simulink model "ctrl_TT_ad_ctrl_cpp_ros_feedback_1"  (R2022b)
settings: Solver=FixedStepAuto  StartTime=0.0  StopTime=Tf  FixedStep=0.05  RelTol=1e-3
StopFcn:
  | save('testdata')
values from neighbouring files (symbols this model uses):
  adap = 1    [testdata.mat]
  Cp = [-70.34790039 18.70597267 -370.8000183 -33.25566673 18.72042656 -369.9571533 3.8263092 17.99342728 -368.5174255 40.77630615 14.78142262 -366.2670288 ... (183 elements, 3x61)]    [testdata.mat]
  Cp_prime = [4.4510680392 0.0017344668 0.1011438 4.44985762706 -0.08575700726 0.1715736104 4.43452754992 -0.37550053768 0.2668049284 4.4276356638 -0.45576590634 0.3213246444 ... (183 elements, 3x61)]    [testdata.mat]
  d = 250    [testdata.mat]
  Kp = 0.1    [testdata.mat]
  L1 =     [testdata.mat]
  Tf = 500    [testdata.mat]
  Ts = 0.05    [testdata.mat]
libraries: robotlib x30, sharedtransform x2, dspmathops x2
settings Model: Creator=yagkim  LastModifiedBy=vpetrov
settings SolverCC: AlgebraicLoopSolver=TrustRegion
settings OptimizationCC: EnhancedBackFolding=on  PassReuseOutputArgsAs=Individual arguments  ZeroExternalMemoryAtStartup=off  ZeroInternalMemoryAtStartup=off  MaxStackSize=64  OptimizeBlockOrder=speed  DifferentSizesBufferReuse=on  OptimizationCustomize=off  EfficientTunableParamExpr=on
settings DebuggingCC: ParameterTunabilityLossMsg=error  UnconnectedInputMsg=warning  UnconnectedOutputMsg=warning  UnconnectedLineMsg=warning  SFMachineParentedDataDiag=warning  ArithmeticOperatorsInVariantConditions=warning
settings HardwareCC: ProdBitPerPointer=32  ProdBitPerSizeT=32  ProdBitPerPtrDiffT=32  ProdLargestAtomicFloat=None  ProdIntDivRoundTo=Undefined  ProdEndianess=Unspecified  ProdWordSize=32  ProdHWDeviceType=Generic->Unspecified (assume 32-bit Generic)
settings ModelReferenceCC: EnableRefExpFcnMdlSchedulingChecks=on
settings SFSimCC: MATLABDynamicMemAlloc=off  CustomCodeUndefinedFunction=UseInterfaceOnly  SimTargetLang=C++
settings RTWCC: Description=Embedded Coder  SystemTargetFile=ert.tlc  HardwareBoard=Robot Operating System (ROS)  TLCOptions="-aInlineSetEventsForThisBaseRateFcn=TLC_FALSE -aSuppressMultiTaskScheduler=TLC_FALSE  -aRateBasedStepFcn=0"  TemplateMakefile=ert_default_tmf  GenerateReport=on  Toolchain=Catkin  LaunchReport=on  TargetLang=C++  DLArmComputeVersion=19.05
settings CodeAppCC: ForceParamTrailComments=on  IgnoreCustomStorageClasses=off  OperatorAnnotations=on  SimulinkDataObjDesc=on  SFDataObjDesc=on  InsertBlockDesc=on
settings ERTTargetCC: SupportContinuousTime=on

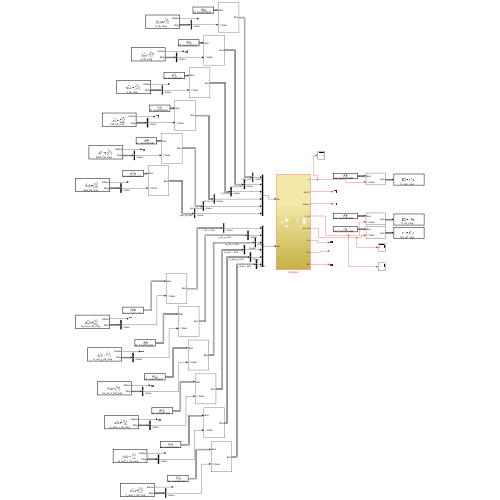
[thumbnail: Simulink's stored preview of the top-level diagram]
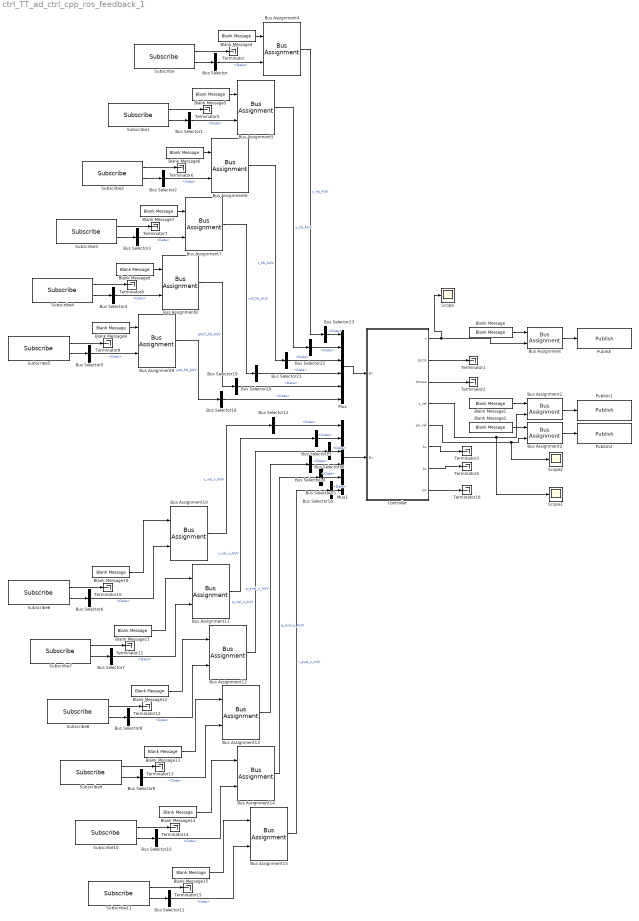
== system ctrl_TT_ad_ctrl_cpp_ros_feedback_1 ==
  Blank Message{,1..2,4..15} (15 alike) : robotlib/Blank Message  messageClass=Message  entityType=std_msgs/Float64  messageType=std_msgs/Float64  SampleTime=inf  legacyBusStruct=off
      settings: LibrarySourceBlock=roslib/ROS/Blank Message
  Bus Assignment{,1..2,4..15} (15 alike) : BusAssignment  AssignedSignals=Data
  Bus Selector{,1..23} (24 alike) : BusSelector  OutputSignals=Data
  Controller : Subsystem
  Mux : Mux  Inputs=6
  Mux1 : Mux  Inputs=6
  Publish : robotlib/Publish  topicSource=Specify your own  topic=/n_rpm_msg  messageType=std_msgs/Float64  legacyBusStruct=off  messageQueueLength=1
      settings: LibrarySourceBlock=roslib/ROS/Publish
  Publish1 : robotlib/Publish  topicSource=Specify your own  topic=/z_ref_msg  messageType=std_msgs/Float64  legacyBusStruct=off  messageQueueLength=1
      settings: LibrarySourceBlock=roslib/ROS/Publish
  Publish2 : robotlib/Publish  topicSource=Specify your own  topic=/psi_ref_msg  messageType=std_msgs/Float64  legacyBusStruct=off  messageQueueLength=1
      settings: LibrarySourceBlock=roslib/ROS/Publish
  Scope : Scope
  Scope1 : Scope
  Scope2 : Scope
  Subscribe : robotlib/Subscribe  topicSource=Specify your own  topic=/x_hb_msg  messageType=std_msgs/Float64  SampleTime=-1  legacyBusStruct=off  messageQueueLength=1
      settings: LibrarySourceBlock=roslib/ROS/Subscribe
  Subscribe1 : robotlib/Subscribe  topicSource=Specify your own  topic=/y_hb_msg  messageType=std_msgs/Float64  SampleTime=-1  legacyBusStruct=off  messageQueueLength=1
      settings: LibrarySourceBlock=roslib/ROS/Subscribe
  Subscribe10 : robotlib/Subscribe  topicSource=Specify your own  topic=/q_avel_y_hb_msg  messageType=std_msgs/Float64  SampleTime=-1  legacyBusStruct=off  messageQueueLength=1
      settings: LibrarySourceBlock=roslib/ROS/Subscribe
  Subscribe11 : robotlib/Subscribe  topicSource=Specify your own  topic=/r_avel_z_hb_msg  messageType=std_msgs/Float64  SampleTime=-1  legacyBusStruct=off  messageQueueLength=1
      settings: LibrarySourceBlock=roslib/ROS/Subscribe
  Subscribe2 : robotlib/Subscribe  topicSource=Specify your own  topic=/z_hb_msg  messageType=std_msgs/Float64  SampleTime=-1  legacyBusStruct=off  messageQueueLength=1
      settings: LibrarySourceBlock=roslib/ROS/Subscribe
  Subscribe3 : robotlib/Subscribe  topicSource=Specify your own  topic=/roll_hb_msg  messageType=std_msgs/Float64  SampleTime=-1  legacyBusStruct=off  messageQueueLength=1
      settings: LibrarySourceBlock=roslib/ROS/Subscribe
  Subscribe4 : robotlib/Subscribe  topicSource=Specify your own  topic=/pitch_hb_msg  messageType=std_msgs/Float64  SampleTime=-1  legacyBusStruct=off  messageQueueLength=1
      settings: LibrarySourceBlock=roslib/ROS/Subscribe
  Subscribe5 : robotlib/Subscribe  topicSource=Specify your own  topic=/yaw_hb_msg  messageType=std_msgs/Float64  SampleTime=-1  legacyBusStruct=off  messageQueueLength=1
      settings: LibrarySourceBlock=roslib/ROS/Subscribe
  Subscribe6 : robotlib/Subscribe  topicSource=Specify your own  topic=/u_vel_x_hb_msg  messageType=std_msgs/Float64  SampleTime=-1  legacyBusStruct=off  messageQueueLength=1
      settings: LibrarySourceBlock=roslib/ROS/Subscribe
  Subscribe7 : robotlib/Subscribe  topicSource=Specify your own  topic=/v_vel_y_hb_msg  messageType=std_msgs/Float64  SampleTime=-1  legacyBusStruct=off  messageQueueLength=1
      settings: LibrarySourceBlock=roslib/ROS/Subscribe
  Subscribe8 : robotlib/Subscribe  topicSource=Specify your own  topic=/w_vel_z_hb_msg  messageType=std_msgs/Float64  SampleTime=-1  legacyBusStruct=off  messageQueueLength=1
      settings: LibrarySourceBlock=roslib/ROS/Subscribe
  Subscribe9 : robotlib/Subscribe  topicSource=Specify your own  topic=/p_avel_x_hb_msg  messageType=std_msgs/Float64  SampleTime=-1  legacyBusStruct=off  messageQueueLength=1
      settings: LibrarySourceBlock=roslib/ROS/Subscribe
  Terminator{,1..16} (17 alike) : Terminator
  wires:
  Bus Assignment4/1 -> Bus Selector23/1  "x_hb_AUV"
  Bus Assignment6/1 -> Bus Selector21/1  "z_hb_AUV"
  Bus Assignment7/1 -> Bus Selector20/1  "roll_hb_AUV"
  Bus Assignment8/1 -> Bus Selector19/1  "pitch_hb_AUV"
  Bus Assignment9/1 -> Bus Selector18/1  "yaw_hb_AUV"
  Mux/1 -> Controller/1(Bx)
  Mux1/1 -> Controller/2(Bv)
  Bus Assignment11/1 -> Bus Selector13/1  "v_vel_y_AUV"
  Bus Assignment12/1 -> Bus Selector17/1  "w_vel_z_AUV"
  Bus Assignment13/1 -> Bus Selector14/1  "p_avel_x_AUV"
  Bus Assignment14/1 -> Bus Selector15/1  "q_avel_y_AUV"
  Bus Assignment15/1 -> Bus Selector16/1  "r_avel_z_AUV"
  Controller/1(n) -> Scope/1, Bus Assignment/2
  Controller/4(z_ref) -> Scope1/1, Bus Assignment1/2
  Controller/5(psi_ref) -> Scope2/1, Bus Assignment2/2
  Controller/6(bv) -> Terminator3/1
  Controller/7(bx) -> Terminator4/1
  Bus Assignment/1 -> Publish/1
  Blank Message/1 -> Bus Assignment/1
  Blank Message1/1 -> Bus Assignment1/1
  Bus Assignment1/1 -> Publish1/1
  Blank Message2/1 -> Bus Assignment2/1
  Bus Assignment2/1 -> Publish2/1
  Subscribe/1 -> Terminator/1
  Bus Selector/1 -> Bus Assignment4/2  "<Data>"
  Subscribe/2 -> Bus Selector/1
  Blank Message4/1 -> Bus Assignment4/1
  Subscribe1/1 -> Terminator5/1
  Bus Selector1/1 -> Bus Assignment5/2  "<Data>"
  Blank Message5/1 -> Bus Assignment5/1
  Subscribe1/2 -> Bus Selector1/1
  Bus Assignment5/1 -> Bus Selector22/1  "y_hb_AUV"
  Blank Message6/1 -> Bus Assignment6/1
  Bus Selector2/1 -> Bus Assignment6/2  "<Data>"
  Subscribe2/2 -> Bus Selector2/1
  Subscribe2/1 -> Terminator6/1
  Blank Message7/1 -> Bus Assignment7/1
  Bus Selector3/1 -> Bus Assignment7/2  "<Data>"
  Subscribe3/2 -> Bus Selector3/1
  Subscribe3/1 -> Terminator7/1
  Blank Message8/1 -> Bus Assignment8/1
  Bus Selector4/1 -> Bus Assignment8/2  "<Data>"
  Subscribe4/2 -> Bus Selector4/1
  Subscribe4/1 -> Terminator8/1
  Bus Selector5/1 -> Bus Assignment9/2  "<Data>"
  Subscribe5/2 -> Bus Selector5/1
  Blank Message9/1 -> Bus Assignment9/1
  Subscribe5/1 -> Terminator9/1
  Bus Selector6/1 -> Bus Assignment10/2  "<Data>"
  Subscribe6/2 -> Bus Selector6/1
  Blank Message10/1 -> Bus Assignment10/1
  Subscribe6/1 -> Terminator10/1
  Bus Assignment10/1 -> Bus Selector12/1  "u_vel_x_AUV"
  Bus Selector7/1 -> Bus Assignment11/2  "<Data>"
  Blank Message11/1 -> Bus Assignment11/1
  Subscribe7/2 -> Bus Selector7/1
  Subscribe7/1 -> Terminator11/1
  Bus Selector8/1 -> Bus Assignment12/2  "<Data>"
  Blank Message12/1 -> Bus Assignment12/1
  Subscribe8/2 -> Bus Selector8/1
  Subscribe8/1 -> Terminator12/1
  Bus Selector9/1 -> Bus Assignment13/2  "<Data>"
  Blank Message13/1 -> Bus Assignment13/1
  Subscribe9/2 -> Bus Selector9/1
  Subscribe9/1 -> Terminator13/1
  Bus Selector10/1 -> Bus Assignment14/2  "<Data>"
  Blank Message14/1 -> Bus Assignment14/1
  Subscribe10/2 -> Bus Selector10/1
  Subscribe10/1 -> Terminator14/1
  Bus Selector11/1 -> Bus Assignment15/2  "<Data>"
  Blank Message15/1 -> Bus Assignment15/1
  Subscribe11/2 -> Bus Selector11/1
  Subscribe11/1 -> Terminator15/1
  Bus Selector12/1 -> Mux1/1  "<Data>"
  Bus Selector13/1 -> Mux1/2  "<Data>"
  Bus Selector14/1 -> Mux1/4  "<Data>"
  Bus Selector15/1 -> Mux1/5  "<Data>"
  Bus Selector16/1 -> Mux1/6  "<Data>"
  Bus Selector17/1 -> Mux1/3  "<Data>"
  Bus Selector18/1 -> Mux/6  "<Data>"
  Bus Selector19/1 -> Mux/5  "<Data>"
  Bus Selector20/1 -> Mux/4  "<Data>"
  Bus Selector21/1 -> Mux/3  "<Data>"
  Bus Selector22/1 -> Mux/2  "<Data>"
  Bus Selector23/1 -> Mux/1  "<Data>"
  Controller/2(dLCG) -> Terminator1/1
  Controller/3(dmass) -> Terminator2/1
  Controller/8(dX) -> Terminator16/1

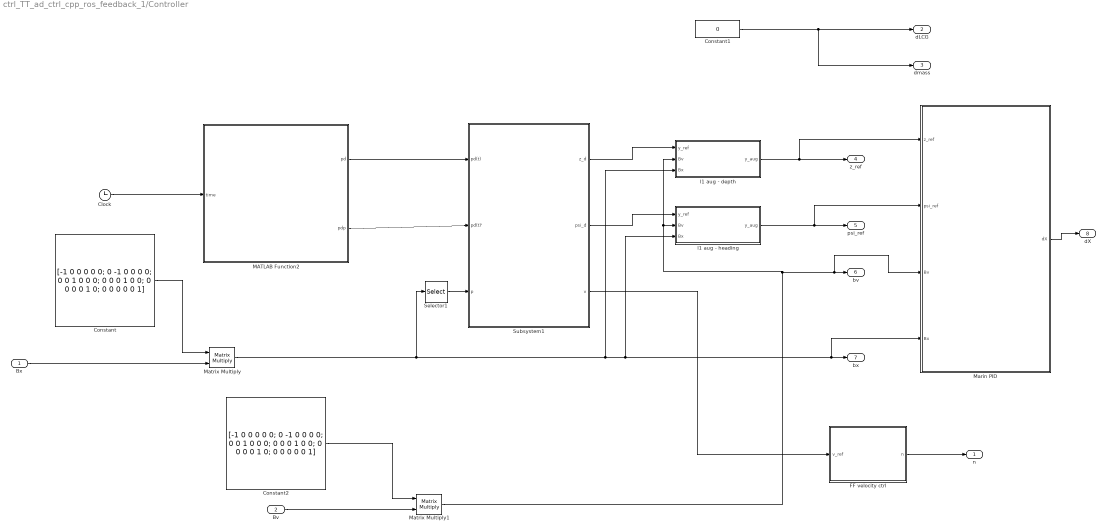
== system ctrl_TT_ad_ctrl_cpp_ros_feedback_1/Controller ==
  Bx : Inport
  Bv : Inport  Port=2
  Clock : Clock
  Constant : Constant  Value=[-1 0 0 0 0 0; 0 -1 0 0 0 0; 0 0 1 0 0 0; 0 0 0 1 0 0; 0 0 0 0 1 0; 0 0 0 0 0 1]
  Constant1 : Constant  Value=0
  Constant2 : Constant  Value=[-1 0 0 0 0 0; 0 -1 0 0 0 0; 0 0 1 0 0 0; 0 0 0 1 0 0; 0 0 0 0 1 0; 0 0 0 0 0 1]
  FF velocity ctrl : MATLAB Function  TreatAsAtomicUnit=on
  MATLAB Function2 : MATLAB Function  TreatAsAtomicUnit=on
  Marin PID : MATLAB Function  TreatAsAtomicUnit=on
  Matrix Multiply : Product  Multiplication=Matrix(*)
  Matrix Multiply1 : Product  Multiplication=Matrix(*)
  Selector1 : Selector  InputPortWidth=6  IndexOptions=Index vector (dialog)  Indices=[1 2 3]  OutputSizes=1
  Subsystem1 : Subsystem
  l1 aug - depth : MATLAB Function  TreatAsAtomicUnit=on
  l1 aug - heading : MATLAB Function  TreatAsAtomicUnit=on
  n : Outport
  dLCG : Outport  Port=2
  dmass : Outport  Port=3
  z_ref : Outport  Port=4
  psi_ref : Outport  Port=5
  bv : Outport  Port=6
  bx : Outport  Port=7
  dX : Outport  Port=8
  wires:
  FF velocity ctrl/1(n) -> n/1
  Subsystem1/3(v) -> FF velocity ctrl/1(v_ref)
  Constant1/1 -> dLCG/1, dmass/1
  MATLAB Function2/1(pd) -> Subsystem1/1(pd(t))
  MATLAB Function2/2(pdp) -> Subsystem1/2(pd(t)')
  Bx/1 -> Matrix Multiply/2
  Selector1/1 -> Subsystem1/3(p)
  Clock/1 -> MATLAB Function2/1(time)
  Matrix Multiply/1 -> Selector1/1, l1 aug - depth/3(Bx), Marin PID/4(Bx), bx/1, l1 aug - heading/3(Bx)
  Constant/1 -> Matrix Multiply/1
  Bv/1 -> Matrix Multiply1/2
  Matrix Multiply1/1 -> l1 aug - depth/2(Bv), l1 aug - heading/2(Bv), Marin PID/3(Bv), bv/1
  Constant2/1 -> Matrix Multiply1/1
  l1 aug - depth/1(y_aug) -> Marin PID/1(z_ref), z_ref/1
  l1 aug - heading/1(y_aug) -> Marin PID/2(psi_ref), psi_ref/1
  Subsystem1/1(z_d) -> l1 aug - depth/1(y_ref)
  Subsystem1/2(psi_d) -> l1 aug - heading/1(y_ref)
  Marin PID/1(dX) -> dX/1

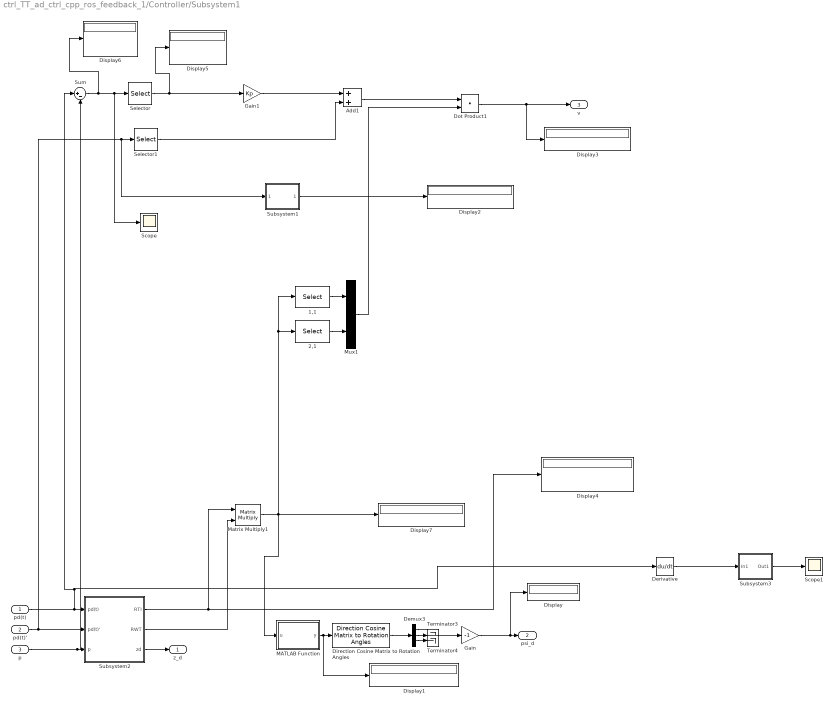
== system ctrl_TT_ad_ctrl_cpp_ros_feedback_1/Controller/Subsystem1 ==
  pd(t) : Inport
  pd(t)' : Inport  Port=2
  p : Inport  Port=3
  1,1 : Selector  NumberOfDimensions=2  InputPortWidth=3  IndexOptions=Index vector (dialog),Index vector (dialog)  Indices=1,1  OutputSizes=1,1
  2,1 : Selector  NumberOfDimensions=2  InputPortWidth=3  IndexOptions=Index vector (dialog),Index vector (dialog)  Indices=2,1  OutputSizes=1,1
  Add1 : Sum
  Demux3 : Demux  Outputs=3
  Derivative : Derivative
  Direction Cosine Matrix to Rotation Angles : sharedtransform/Direction Cosine Matrix to Rotation Angles  rotationOrder=ZYX  aMode=aMode  action=None  tolerance=eps(2)
      settings: LibrarySourceBlock=|
      | aerolibtransform2/Direction Cosine Matrix
      | to Rotation Angles
  Display{,1..7} (8 alike) : Display
  Dot Product1 : DotProduct  OutDataTypeStr=Inherit: Inherit via internal rule
  Gain : Gain  Gain=-1
  Gain1 : Gain  Gain=Kp
  MATLAB Function : MATLAB Function  TreatAsAtomicUnit=on
  Matrix Multiply1 : Product  Multiplication=Matrix(*)
  Mux1 : Mux  Inputs=2
  Scope : Scope
  Scope1 : Scope
  Selector : Selector  InputPortWidth=3  IndexOptions=Index vector (dialog)  Indices=[1 2]  OutputSizes=1
  Selector1 : Selector  InputPortWidth=3  IndexOptions=Index vector (dialog)  Indices=[1 2]  OutputSizes=1
  Subsystem1 : Subsystem
  Subsystem2 : Subsystem
  Subsystem3 : Subsystem
  Sum : Sum  Inputs=|+-
  Terminator3 : Terminator
  Terminator4 : Terminator
  z_d : Outport
  psi_d : Outport  Port=2
  v : Outport  Port=3
  wires:
  pd(t)'/1 -> Subsystem2/2(pd(t)'), Subsystem1/1(pd(t)'), Selector1/1
  pd(t)/1 -> Derivative/1, Sum/1, Subsystem2/1(pd(t))
  p/1 -> Sum/2, Subsystem2/3(p)
  Subsystem2/1(RTI) -> Matrix Multiply1/1, Display4/1
  2,1/1 -> Mux1/2
  1,1/1 -> Mux1/1
  Subsystem2/3(zd) -> z_d/1
  Gain/1 -> Display/1, psi_d/1
  Subsystem2/2(RWT) -> Matrix Multiply1/2
  Sum/1 -> Display6/1, Scope/1, Selector/1
  Derivative/1 -> Subsystem3/1(In1)
  Subsystem3/1(Out1) -> Scope1/1
  Gain1/1 -> Add1/1
  Add1/1 -> Dot Product1/1
  Mux1/1 -> Dot Product1/2
  Dot Product1/1 -> Display3/1, v/1
  Selector/1 -> Display5/1, Gain1/1
  Selector1/1 -> Add1/2
  Subsystem1/1(Out1) -> Display2/1
  Direction Cosine Matrix to Rotation Angles/1 -> Demux3/1
  Matrix Multiply1/1 -> MATLAB Function/1(u), Display7/1, 2,1/1, 1,1/1
  MATLAB Function/1(y) -> Display1/1, Direction Cosine Matrix to Rotation Angles/1
  Demux3/2 -> Terminator3/1
  Demux3/3 -> Terminator4/1
  Demux3/1 -> Gain/1

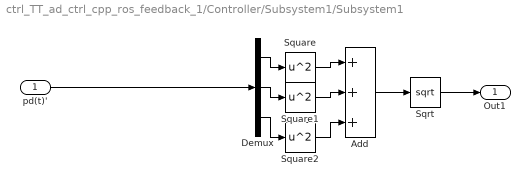
== system ctrl_TT_ad_ctrl_cpp_ros_feedback_1/Controller/Subsystem1/Subsystem1 ==
  pd(t)' : Inport
  Add : Sum  Inputs=+++
  Demux : Demux  Outputs=3
  Sqrt : Sqrt
  Square : Math  Operator=square
  Square1 : Math  Operator=square
  Square2 : Math  Operator=square
  Out1 : Outport
  wires:
  Square2/1 -> Add/3
  Demux/3 -> Square2/1
  pd(t)'/1 -> Demux/1
  Demux/1 -> Square/1
  Demux/2 -> Square1/1
  Add/1 -> Sqrt/1
  Square/1 -> Add/1
  Square1/1 -> Add/2
  Sqrt/1 -> Out1/1

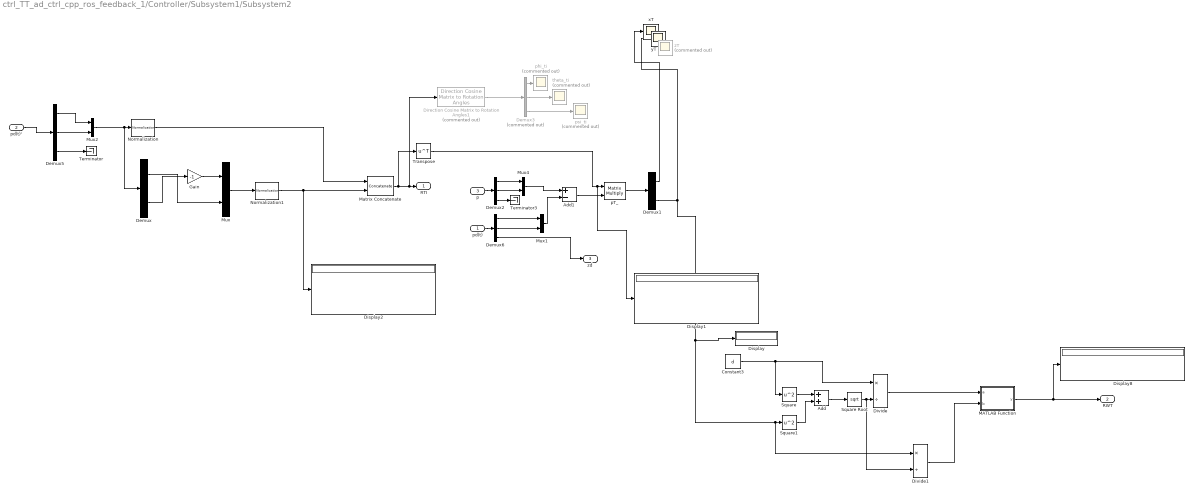
== system ctrl_TT_ad_ctrl_cpp_ros_feedback_1/Controller/Subsystem1/Subsystem2 ==
  pd(t) : Inport
  pd(t)' : Inport  Port=2
  p : Inport  Port=3
  Add : Sum
  Add1 : Sum  Inputs=+-
  Constant3 : Constant  Value=d
  Demux : Demux  Outputs=2
  Demux1 : Demux  Outputs=2
  Demux2 : Demux  Outputs=3
  Demux3 : Demux  Commented=on  Outputs=3
  Demux5 : Demux  Outputs=3
  Demux6 : Demux  Outputs=3
  Direction Cosine Matrix to Rotation Angles1 : sharedtransform/Direction Cosine Matrix to Rotation Angles  Commented=on  rotationOrder=XYZ  aMode=aMode  action=None  tolerance=eps(2)
  Display{,1..2,8} (4 alike) : Display
  Divide : Product  Inputs=*/
  Divide1 : Product  Inputs=*/
  Gain : Gain  Gain=-1
  MATLAB Function : MATLAB Function  TreatAsAtomicUnit=on
  Matrix Concatenate : Concatenate  Mode=Multidimensional array  ConcatenateDimension=2
  Mux{,1..2,4} (4 alike) : Mux  Inputs=2
  Normalization : dspmathops/Normalization  NormType=2-norm  Bias=1e-10  NormOver=Each column  Dimension=1  roundingMode=Floor  overflowMode=off  accumDataTypeStr=Inherit: Same as product output  accumLastDataTypeStr=Inherit: Same as product output  outputDataTypeStr=Inherit: Same as product output  outputMin=[]  outputMax=[]  outputLastDataTypeStr=Inherit: Same as product output
  Normalization1 : dspmathops/Normalization  NormType=2-norm  Bias=1e-10  NormOver=Each column  Dimension=1  roundingMode=Floor  overflowMode=off  accumDataTypeStr=Inherit: Same as product output  accumLastDataTypeStr=Inherit: Same as product output  outputDataTypeStr=Inherit: Same as product output  outputMin=[]  outputMax=[]  outputLastDataTypeStr=Inherit: Same as product output
  Square : Math  Operator=square
  Square Root : Sqrt
  Square1 : Math  Operator=square
  Terminator : Terminator
  Terminator3 : Terminator
  Transpose : Math  Operator=transpose
  pT_ : Product  Multiplication=Matrix(*)
  phi_ti : Scope  Commented=on
  psi_ti : Scope  Commented=on
  theta_ti : Scope  Commented=on
  xT : Scope
  yT : Scope
  zT : Scope  Commented=on
  RTI : Outport
  RWT : Outport  Port=2
  zd : Outport  Port=3
  wires:
  Gain/1 -> Mux/1
  Demux/2 -> Gain/1
  Demux/1 -> Mux/2
  Mux/1 -> Normalization1/1
  Normalization/1 -> Matrix Concatenate/1
  Normalization1/1 -> Matrix Concatenate/2, Display2/1
  Matrix Concatenate/1 -> Direction Cosine Matrix to Rotation Angles1/1, RTI/1, Transpose/1
  Transpose/1 -> Display1/1, pT_/1
  Add1/1 -> pT_/2
  pT_/1 -> Demux1/1
  Demux1/2 -> yT/1, Display/1, Divide1/1, Square1/1
  Demux1/1 -> xT/1
  Direction Cosine Matrix to Rotation Angles1/1 -> Demux3/1
  Demux3/3 -> psi_ti/1
  Demux3/2 -> theta_ti/1
  Demux3/1 -> phi_ti/1
  Constant3/1 -> Square/1, Divide/1
  Square Root/1 -> Divide1/2, Divide/2
  Add/1 -> Square Root/1
  Square/1 -> Add/1
  Square1/1 -> Add/2
  Divide/1 -> MATLAB Function/1(a)
  Divide1/1 -> MATLAB Function/2(b)
  MATLAB Function/1(y) -> RWT/1, Display8/1
  Demux6/3 -> zd/1
  pd(t)'/1 -> Demux5/1
  Mux2/1 -> Demux/1, Normalization/1
  Demux5/1 -> Mux2/1
  Demux5/2 -> Mux2/2
  Demux5/3 -> Terminator/1
  Demux2/1 -> Mux4/1
  Demux2/3 -> Terminator3/1
  Demux2/2 -> Mux4/2
  Mux4/1 -> Add1/1
  p/1 -> Demux2/1
  Demux6/1 -> Mux1/1
  Demux6/2 -> Mux1/2
  pd(t)/1 -> Demux6/1
  Mux1/1 -> Add1/2

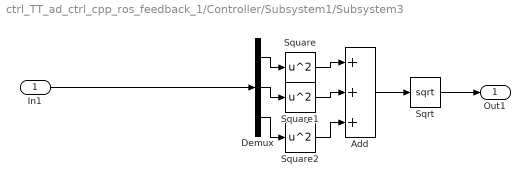
== system ctrl_TT_ad_ctrl_cpp_ros_feedback_1/Controller/Subsystem1/Subsystem3 ==
  In1 : Inport
  Add : Sum  Inputs=+++
  Demux : Demux  Outputs=3
  Sqrt : Sqrt
  Square : Math  Operator=square
  Square1 : Math  Operator=square
  Square2 : Math  Operator=square
  Out1 : Outport
  wires:
  Sqrt/1 -> Out1/1
  Square1/1 -> Add/2
  Square/1 -> Add/1
  Add/1 -> Sqrt/1
  Demux/2 -> Square1/1
  Demux/1 -> Square/1
  In1/1 -> Demux/1
  Demux/3 -> Square2/1
  Square2/1 -> Add/3

== matlab function ctrl_TT_ad_ctrl_cpp_ros_feedback_1/Controller/FF velocity ctrl ==
  settings: updateMethod=DISCRETE
  data: v_ref input; n output
function n   = fcn(v_ref)




KP_n = 5;
FF_inv = 4;



%% Prop
n = v_ref/FF_inv;

== matlab function ctrl_TT_ad_ctrl_cpp_ros_feedback_1/Controller/l1 aug - heading ==
  settings: updateMethod=DISCRETE
  data: y_ref input; Bv input; Bx input; y_aug output; Ts parameter; adap parameter; L1 parameter
function y_aug    = fcn(y_ref,Bv,Bx,Ts,adap,L1)
%pd,NomegaNI,

persistent xu xd


%% Variables for feedback
x = Bx(1); y = Bx(2); z = Bx(3); phi = Bx(4); theta = Bx(5); psi = Bx(6);
p = [x;y;z];
uN = Bv(1); vN = Bv(2); wN = Bv(3); pB = Bv(4); qB=Bv(5); rB = Bv(6);
uB = -uN; vB = -vN; wB = wN;

%% Control Parameters  
% Gains for PF augmentation
Ts = Ts;
Am = L1.Amz; Bm = L1.Bmz; Cm = L1.Cmz; 
Phiinv = L1.Phiinvz; Lambda = L1.Lambdaz;
Ao = L1.Aoz; Bo = L1.Boz; Co = L1.Coz;

%% Output Definition
y = psi;;

%% Initialize
if isempty(xu)
        xu = zeros(length(Ao),1);
        xd = Cm'*inv(Cm*Cm')*y;
        xu_next = xu;
        xd_next = xd;
end



%% L1 Augmentation - dive

if adap 

    yd = Cm*xd;
    vec1    =   [eye(size(Bm,2)); zeros(size(Am,1)-size(Bm,2),size(Bm,2))];
    sigma = -Phiinv*expm(Lambda*(Am/Lambda)*Ts)*vec1*(yd-y);

    xu_next = expm(Ao*Ts)*xu + inv(Ao)*(expm(Ao*Ts)-eye(length(Bo)))*(Bo*expm(-Am*Ts)*sigma);
    Kg = -inv(Cm*inv(Am)*Bm);
    ud = Kg*y_ref - Co*xu;

    xd_next = expm(Am*Ts)*xd + inv(Am)*(expm(Am*Ts)-eye(length(Am)))*(Bm*ud + sigma);

    y_aug = ud;

else 

    y_aug = y_ref;

    xd_next = xd;
    xu_next = xu;

end




%% Save variables for next loop
xu = xu_next;
xd = xd_next;

== matlab function ctrl_TT_ad_ctrl_cpp_ros_feedback_1/Controller/l1 aug - depth ==
  settings: updateMethod=DISCRETE
  data: y_ref input; Bv input; Bx input; y_aug output; Ts parameter; adap parameter; L1 parameter
function y_aug    = fcn(y_ref,Bv,Bx,Ts,adap,L1)
%pd,NomegaNI,

persistent xu xd


%% Variables for feedback
x = Bx(1); y = Bx(2); z = Bx(3); phi = Bx(4); theta = Bx(5); psi = Bx(6);
p = [x;y;z];
uN = Bv(1); vN = Bv(2); wN = Bv(3); pB = Bv(4); qB=Bv(5); rB = Bv(6);
uB = -uN; vB = -vN; wB = wN;

%% Control Parameters  
% Gains for PF augmentation
Ts = Ts;
Am = L1.Amz; Bm = L1.Bmz; Cm = L1.Cmz; 
Phiinv = L1.Phiinvz; Lambda = L1.Lambdaz;
Ao = L1.Aoz; Bo = L1.Boz; Co = L1.Coz;
%% Output Definition
y = z; 

%% Initialize
if isempty(xu)
        xu = zeros(length(Ao),1);
        xd = Cm'*inv(Cm*Cm')*y;
        xu_next = xu;
        xd_next = xd;
end



%% L1 Augmentation - dive

if adap 

    yd = Cm*xd;
    vec1    =   [eye(size(Bm,2)); zeros(size(Am,1)-size(Bm,2),size(Bm,2))];
    sigma = -Phiinv*expm(Lambda*(Am/Lambda)*Ts)*vec1*(yd-y);

    xu_next = expm(Ao*Ts)*xu + inv(Ao)*(expm(Ao*Ts)-eye(length(Bo)))*(Bo*expm(-Am*Ts)*sigma);
    Kg = -inv(Cm*inv(Am)*Bm);
    ud = Kg*y_ref - Co*xu;

    xd_next = expm(Am*Ts)*xd + inv(Am)*(expm(Am*Ts)-eye(length(Am)))*(Bm*ud + sigma);

    y_aug = ud;

else 

    y_aug = y_ref;

    xd_next = xd;
    xu_next = xu;

end




%% Save variables for next loop
xu = xu_next;
xd = xd_next;

== matlab function ctrl_TT_ad_ctrl_cpp_ros_feedback_1/Controller/Subsystem1/MATLAB Function ==
  data: u input; y output
function y = R3(u)

y = [u(1,1) u(1,2) 0; u(2,1) u(2,2) 0; 0 0 1];

== matlab function ctrl_TT_ad_ctrl_cpp_ros_feedback_1/Controller/MATLAB Function2 ==
  data: time input; pd output; pdp output; Cp_prime parameter; Cp parameter; Tf parameter
function [pd, pdp] = fcn(time, Cp_prime, Cp, Tf)




pd = BernsteinPoly(Cp,time,0,Tf);
pdp = BernsteinPoly(Cp_prime,time,0,Tf);

% pd = [gamma; gamma/2 ; -50];
% 
% 
% pdp = [1 ; 1/2; 0];

end










function  poly_t  = BernsteinPoly(Cp,t,t0,tf)

% INPUTS:
% Cp is a matrix n by N+1 (n: dimension of polynomial, N: order of polynomial) 
% t is a time vector
% OUTPUT:
% poly_t: n-dimensional polynomial evaluated at each time t

% if t is a scalar, it returns the value of Bernstein Poly at t in [t0,tf]
% if t0 and tf are not provided, it returns the value of Bernstein Poly at t in [0,1]

% Written by: Venanzio Cichella       

%%%%%%%%%%%%%%%%%%%%%%%%%%%%%%%%%%%%%%%%%%%%%%

coder.extrinsic('exist')

[~, N] = size(Cp);
N = N-1;


% if length(t) > 1
%     B = BernsteinMatrix_a2b(N,t)';
%     poly_t = Cp*B;
% else
%     if ~exist('t0','var')
%         B = BernsteinMatrix_a2b(N,t)';
%         poly_t = Cp*B;
%     else
%         B = BernsteinMatrix_a2b(N,t,t0,tf)';
%         poly_t = Cp*B;
%     end
% end
B = BernsteinMatrix_a2b(N,t,t0,tf)';
poly_t = Cp*B;


end










function b = BernsteinMatrix_a2b(N, t, tmin, tmax)

% Inputs: order N, time vector t = [t0 ... tm], no need for tmin and tmax.
% Output: b = [b0N(t0) b1N(t0) ... bNN(t0);
%              b0N(t1) b1N(t1) ... bNN(t1);
%              ...
%              b0N(tm) b1N(tm) ... bNN(tm);
% Use: If Cp is a row vector of N+1 control points,
%       the Nth order Bezier curve is given by xN=Cp*b';
% This function is used in BernsteinPoly

% Alternatively
% Inputs: order n, scalar time t', tmin and tmax
% Output: b = [b0n(t') b1n(t') ... bnn(t')]
% Use: If Cp is a row vector of N+1 control points,
%       the Nth order Bezier curve evaluated at t' is given by xn=Cp*b';
% Comment: This is more efficient but not as robust as de Casteljau
%           It works best for low-order curves

% Written by: Venanzio Cichella       

%%%%%%%%%%%%%%%%%%%%%%%%%%%%%%%%%%%%%%%%%%%%%%

if length(t) > 1
    tmax = t(length(t));
    tmin = t(1);
end
%coder.extrinsic('exist')
%if ~exist('tmin','var')
%    tmin = 0; tmax = 1;
%end



% compute B(j+1) = binomial(n, j), j = 0..n
t = t';
B = ones(N+1, 1); 
for j = 1:ceil(N/2)
  B(j+1) = B(j)*(N+1-j)/j;
  B(N+1-j) = B(j+1);
end
% compute T(i, j) = (t(i)-tmin)^j, TT(i, j) = (tmax-t(i))^(N-j)
T = ones(length(t), N+1);
TT = ones(length(t), N+1);
% turn a row t into a column t so that 
% we can do diag(t)*T(:,j) by t.*T(:,j)
tp = reshape(t, length(t), 1)-tmin;
ttp = tmax - t;
% Compute binomial(N, j)*(t(i)-tmin)^j*(tmax-t(i))^(N-j)
for j = 1:N 
  T(:, j+1) = tp .* T(:, j); 
  T(:, j) = T(:, j) .* B(j);
 TT(:,N+1-j) = ttp .* TT(:,N+2-j);
end

% Compute binomial(N, j)*(t(i)-tmin)^j*(tmax-t(i))^(N-j)/((tmax-tmin)^N)
b =  T.*TT./((tmax-tmin)^N);

end

== matlab function ctrl_TT_ad_ctrl_cpp_ros_feedback_1/Controller/Subsystem1/Subsystem2/MATLAB Function ==
  data: a input; y output; b input
function y = fcn(a,b)

%y = [a,b,0;-b,a,0;0,0,1];
y = [a,b;-b,a];

== matlab function ctrl_TT_ad_ctrl_cpp_ros_feedback_1/Controller/Marin PID ==
  settings: updateMethod=DISCRETE
  data: z_ref input; psi_ref input; Bv input; Bx input; dX output; Ts parameter
function dX   = fcn(z_ref,psi_ref,Bv,Bx,Ts)

persistent zerr_prev zerr_int_prev thetaerr_prev thetaerr_int_prev psierr_prev psierr_int_prev

%% Initialize
if isempty(zerr_prev)
        zerr_prev = 0;
        zerr_int_prev = 0;
        thetaerr_prev = 0;
        thetaerr_int_prev = 0;
        psierr_prev = 0;
        psierr_int_prev = 0;
end


%% Variables for feedback
x = Bx(1); y = Bx(2); z = Bx(3); phi = Bx(4); theta = Bx(5); psi = Bx(6);
p = [x;y;z];
uN = Bv(1); vN = Bv(2); wN = Bv(3); pB = Bv(4); qB=Bv(5); rB = Bv(6);
uB = -uN; vB = -vN; wB = wN;


%% Gains
KP_APz = 3;
KI_APz = 0*0.1044;
KD_APz = 3;

KP_APtheta = 3;
KI_APtheta = 0*0.1466;
KD_APtheta = 3;

KP_APpsi = 3;
KI_APpsi = 0;
KD_APpsi = 12.199;








%% Autopilot (depth)
zerr = z_ref - z;
zerrint = zerr*Ts+zerr_int_prev;
zerrdot = (zerr-zerr_prev)/Ts;
dvz = KP_APz*zerr+KI_APz*zerrint+KD_APz*zerrdot;

theta_ref = 0;
thetaerr = (theta_ref - theta)*180/pi;
thetaerrint = thetaerr*Ts+thetaerr_int_prev;
thetaerrdot = (thetaerr-thetaerr_prev)/Ts;
dvtheta = KP_APtheta*thetaerr+KI_APtheta*thetaerrint+KD_APtheta*thetaerrdot;

dv = dvz + dvtheta;

%% Autopilot (yaw)
psierr = (psi_ref - psi)*180/pi;
psierrint = psierr*Ts+psierr_int_prev;
psierrdot = (psierr-psierr_prev)/Ts;
dh = KP_APpsi*psierr+KI_APpsi*psierrint+KD_APpsi*psierrdot;


%% Control Allocation
d1 = -dv+dh; 
d2 = -dv-dh; 
d3 = dv-dh; 
d4 = dv+dh; 
d5 = dv; 
dX = [d1 ; d2 ; d3 ; d4 ; d5];





%% Save variables for next loop
zerr_prev = zerr;
zerr_int_prev = zerrint;
thetaerr_prev = thetaerr;
thetaerr_int_prev = thetaerrint;
psierr_prev = psierr;
psierr_int_prev = psierrint;
